simulink model "model_only_GD_constant_muscle_admittance_aug_gain"  (R2020a)
settings: Solver=FixedStepAuto  StartTime=0.0  StopTime=180  FixedStep=0.002  RelTol=1e-6  EnableMultiTasking=on
libraries: dspmtrx3 x1
settings Model: SimulationMode=accelerator  Creator=Tenghu  LastModifiedBy=ripme
settings DataIOCC: SaveFormat=Array  SignalLoggingSaveFormat=ModelDataLogs  SaveOutput=off  ReturnWorkspaceOutputs=off
settings OptimizationCC: ExpressionDepthLimit=2147483647  EfficientMapNaN2IntZero=off  LifeSpan=inf
settings DebuggingCC: UnderspecifiedInitializationDetection=Classic  MergeDetectMultiDrivingBlocksExec=none  SolverPrmCheckMsg=warning  FcnCallInpInsideContextMsg=warning  StateNameClashWarn=warning  SFUnexpectedBacktrackingDiag=warning  SFNoUnconditionalDefaultTransitionDiag=warning  SFExecutionAtInitializationDiag=none  UnderSpecifiedDimensionMsg=warning  ArithmeticOperatorsInVariantConditions=warning
settings HardwareCC: ProdBitPerPointer=32  ProdBitPerSizeT=32  ProdBitPerPtrDiffT=32  ProdLargestAtomicFloat=None  ProdIntDivRoundTo=Undefined  ProdEndianess=Unspecified  ProdWordSize=32  ProdHWDeviceType=32-bit Generic  TargetBitPerPointer=64  TargetBitPerSizeT=64  TargetBitPerPtrDiffT=64  TargetLongLongMode=on  TargetIntDivRoundTo=Zero  TargetEndianess=LittleEndian  TargetWordSize=64  TargetHWDeviceType=MATLAB Host  ProdEqTarget=off
settings ModelReferenceCC: PropagateSignalLabelsOutOfModel=off
settings SFSimCC: SimUseLocalCustomCode=off  SimParseCustomCode=off  CustomCodeUndefinedFunction=UseInterfaceOnly
settings CodeAppCC: MaxIdLength=128
settings GRTTargetCC: TargetLangStandard=C89/C90 (ANSI)  CombineOutputUpdateFcns=off  GRTInterface=on
settings ConfigComp: CovMetricSettings=dw  CovHtmlReporting=on  CovSaveCumulativeToWorkspaceVar=on  CovSaveSingleToWorkspaceVar=on  CovExternalEMLEnable=off

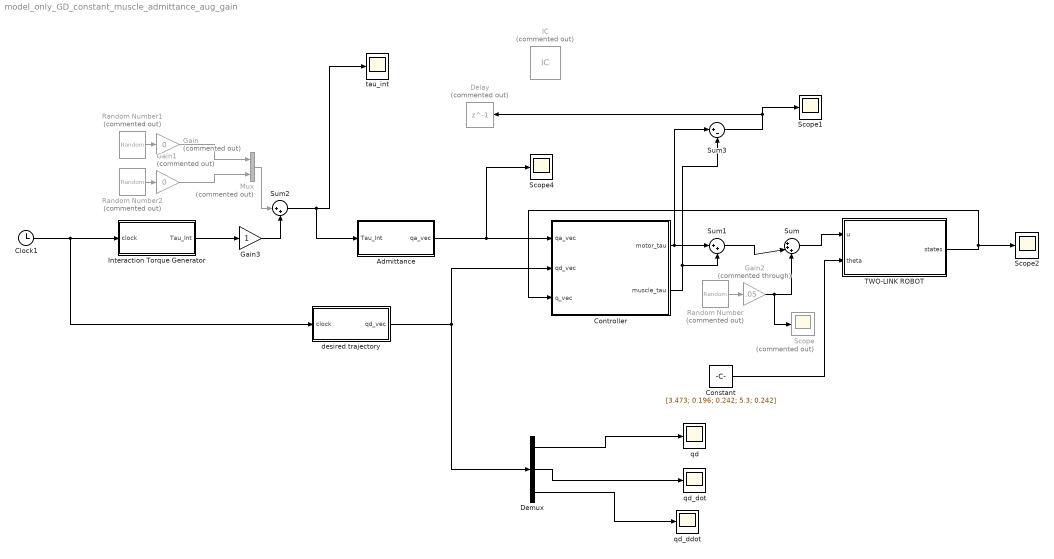
== system model_only_GD_constant_muscle_admittance_aug_gain ==
  Admittance : Subsystem
  Clock1 : Clock
  Constant : Constant  Value=|
      | [3.473;
      | 0.196;
      | 0.242; 5.3; 0.242]
  Controller : Subsystem
  Delay : Delay  Commented=on  DelayLength=1  InitialCondition=[0;0]
  Demux : Demux  Outputs=3
  Gain : Gain  Commented=on  Gain=0
  Gain1 : Gain  Commented=on  Gain=0
  Gain2 : Gain  Commented=through  Gain=.05
  Gain3 : Gain
  IC : InitialCondition  Commented=on  Value=[0;0]
  Interaction Torque Generator : Subsystem
  Mux : Mux  Commented=on  Inputs=2
  Random Number : RandomNumber  Commented=on  Mean=5  SampleTime=0.002
  Random Number1 : RandomNumber  Commented=on  Mean=1  Variance=.5  SampleTime=0.002
  Random Number2 : RandomNumber  Commented=on  Mean=1  Variance=.2  SampleTime=0.002
  Scope : Scope  Commented=on
  Scope1 : Scope
  Scope2 : Scope
  Scope4 : Scope
  Sum : Sum  Inputs=|+++
  Sum1 : Sum  Inputs=|++
  Sum2 : Sum  Inputs=|++
  Sum3 : Sum  Inputs=|+-
  TWO-LINK ROBOT : Subsystem
  desired trajectory : Subsystem
  qd : Scope
  qd_ddot : Scope
  qd_dot : Scope
  tau_int : Scope
  wires:
  TWO-LINK ROBOT/1(states) -> Scope2/1, Controller/3(q_vec)
  Sum/1 -> TWO-LINK ROBOT/1(u)
  Clock1/1 -> Interaction Torque Generator/1(clock), desired trajectory/1(clock)
  desired trajectory/1(qd_vec) -> Controller/2(qd_vec), Demux/1
  Admittance/1(qa_vec) -> Scope4/1, Controller/1(qa_vec)
  Controller/1(motor_tau) -> Sum3/1, Sum1/1
  Sum1/1 -> Sum/2
  Sum2/1 -> Admittance/1("Tau_Int "), tau_int/1
  Mux/1 -> Sum2/1
  Random Number1/1 -> Gain/1
  Random Number2/1 -> Gain1/1
  Gain1/1 -> Mux/2
  Gain/1 -> Mux/1
  Random Number/1 -> Gain2/1
  Gain2/1 -> Sum/3, Scope/1
  Controller/2(muscle_tau) -> Sum1/2, Sum3/2
  Sum3/1 -> Scope1/1, Delay/1
  Gain3/1 -> Sum2/2
  Interaction Torque Generator/1(Tau_Int) -> Gain3/1
  Demux/1 -> qd/1
  Demux/2 -> qd_dot/1
  Demux/3 -> qd_ddot/1
  Constant/1 -> TWO-LINK ROBOT/2(theta)

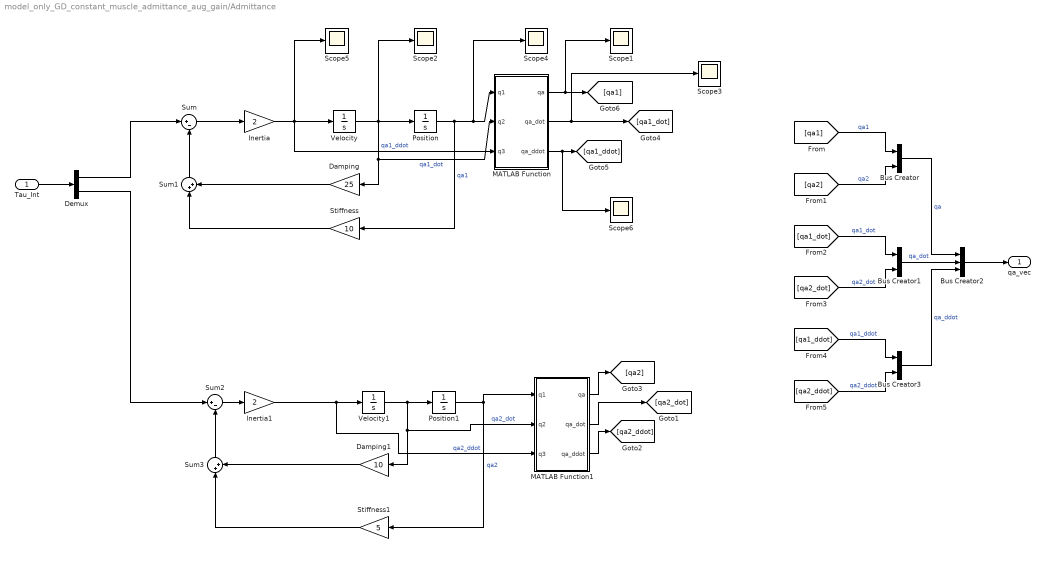
== system model_only_GD_constant_muscle_admittance_aug_gain/Admittance ==
  "Tau_Int " : Inport
  Bus Creator : BusCreator  Inputs=2
  Bus Creator1 : BusCreator  Inputs=2
  Bus Creator2 : BusCreator  Inputs=3
  Bus Creator3 : BusCreator  Inputs=2
  Damping : Gain  Gain=25
  Damping1 : Gain  Gain=10
  Demux : Demux  Outputs=2
  Inertia : Gain  Gain=2
  Inertia1 : Gain  Gain=2
  MATLAB Function : MATLAB Function  TreatAsAtomicUnit=on
  MATLAB Function1 : MATLAB Function  TreatAsAtomicUnit=on
  Position : Integrator
  Position1 : Integrator
  Scope{1..6} (6 alike) : Scope
  Stiffness : Gain  Gain=10
  Stiffness1 : Gain  Gain=5
  Sum : Sum  Inputs=|+-
  Sum1 : Sum  Inputs=|++
  Sum2 : Sum  Inputs=|+-
  Sum3 : Sum  Inputs=|++
  Velocity : Integrator
  Velocity1 : Integrator
  qa_vec : Outport  VectorParamsAs1DForOutWhenUnconnected=off
  wires:
  Inertia/1 -> MATLAB Function/3(q3), Scope5/1, Velocity/1  "qa1_ddot"
  Sum/1 -> Inertia/1
  Sum1/1 -> Sum/2
  Velocity/1 -> MATLAB Function/2(q2), Damping/1, Scope2/1, Position/1  "qa1_dot"
  Damping/1 -> Sum1/2
  Stiffness/1 -> Sum1/1
  Position/1 -> Scope4/1, MATLAB Function/1(q1), Stiffness/1  "qa1"
  "Tau_Int "/1 -> Demux/1
  Demux/1 -> Sum/1
  Velocity1/1 -> Position1/1, MATLAB Function1/2(q2), Damping1/1  "qa2_dot"
  Inertia1/1 -> MATLAB Function1/3(q3), Velocity1/1  "qa2_ddot"
  Position1/1 -> MATLAB Function1/1(q1), Stiffness1/1  "qa2"
  Sum2/1 -> Inertia1/1
  Damping1/1 -> Sum3/2
  Demux/2 -> Sum2/1
  Sum3/1 -> Sum2/2
  Stiffness1/1 -> Sum3/1
  [qa1] -> Bus Creator/1  "qa1"
  [qa2] -> Bus Creator/2  "qa2"
  [qa1_dot] -> Bus Creator1/1  "qa1_dot"
  [qa2_dot] -> Bus Creator1/2  "qa2_dot"
  Bus Creator1/1 -> Bus Creator2/2  "qa_dot"
  Bus Creator/1 -> Bus Creator2/1  "qa"
  [qa1_ddot] -> Bus Creator3/1  "qa1_ddot"
  [qa2_ddot] -> Bus Creator3/2  "qa2_ddot"
  Bus Creator3/1 -> Bus Creator2/3  "qa_ddot"
  Bus Creator2/1 -> qa_vec/1
  MATLAB Function/1(qa) -> Scope1/1, [qa1]
  MATLAB Function/2(qa_dot) -> [qa1_dot], Scope3/1
  MATLAB Function/3(qa_ddot) -> Scope6/1, [qa1_ddot]
  MATLAB Function1/1(qa) -> [qa2]
  MATLAB Function1/3(qa_ddot) -> [qa2_ddot]
  MATLAB Function1/2(qa_dot) -> [qa2_dot]

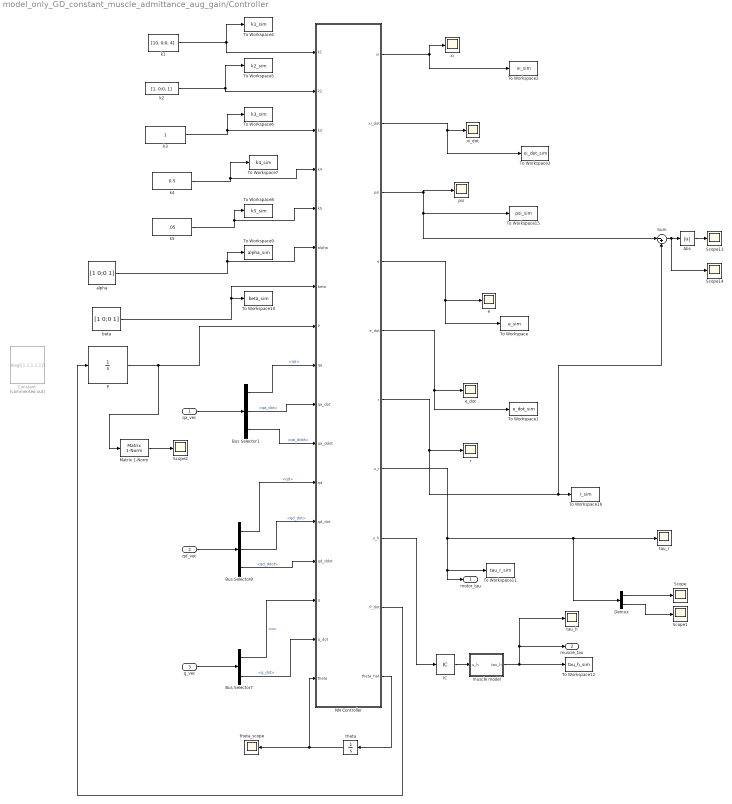
== system model_only_GD_constant_muscle_admittance_aug_gain/Controller ==
  qa_vec : Inport
  qd_vec : Inport  Port=2
  q_vec : Inport  Port=3
  Abs : Abs
  Bus Selector1 : BusSelector  OutputSignals=qa,qa_dot,qa_ddot
  Bus Selector7 : BusSelector  OutputSignals=q,q_dot
  Bus Selector8 : BusSelector  OutputSignals=qd,qd_dot,qd_ddot
  Constant : Constant  Commented=on  Value=diag([1,1,1,1,1])
  Demux : Demux  Outputs=2
  IC : InitialCondition  Value=[0;0]
  Matrix 1-Norm : dspmtrx3/Matrix  1-Norm  roundingMode=Floor  overflowMode=off  outputDataTypeStr=Inherit: Same as accumulator  outputMin=[]  outputMax=[]  outputLastDataTypeStr=Inherit: Same as accumulator
      settings: SourceProductBaseCode=DS
  "NN Controller " : MATLAB Function  TreatAsAtomicUnit=on
  P : Integrator  InitialCondition=diag([1,1,1,1,1]*5)
  Scope{,1..2,13..14} (5 alike) : Scope
  Sum : Sum  Inputs=|-+
  To Workspace : ToWorkspace  VariableName=e_sim  SaveFormat=Timeseries  SampleTime=-1
  To Workspace1 : ToWorkspace  VariableName=e_dot_sim  SaveFormat=Timeseries  SampleTime=-1
  To Workspace10 : ToWorkspace  VariableName=beta_sim  SaveFormat=Timeseries  SampleTime=-1
      settings: MaxDataPoints=1
  To Workspace11 : ToWorkspace  VariableName=tau_r_sim  SaveFormat=Timeseries  SampleTime=-1
  To Workspace12 : ToWorkspace  VariableName=tau_h_sim  SaveFormat=Timeseries  SampleTime=-1
  To Workspace15 : ToWorkspace  VariableName=psi_sim  SaveFormat=Timeseries  SampleTime=-1
  To Workspace16 : ToWorkspace  VariableName=r_sim  SaveFormat=Timeseries  SampleTime=-1
  To Workspace2 : ToWorkspace  VariableName=xi_sim  SaveFormat=Timeseries  SampleTime=-1
  To Workspace3 : ToWorkspace  VariableName=xi_dot_sim  SaveFormat=Timeseries  SampleTime=-1
  To Workspace4 : ToWorkspace  VariableName=k1_sim  SaveFormat=Timeseries  SampleTime=-1
      settings: MaxDataPoints=1
  To Workspace5 : ToWorkspace  VariableName=k2_sim  SaveFormat=Timeseries  SampleTime=-1
      settings: MaxDataPoints=1
  To Workspace6 : ToWorkspace  VariableName=k3_sim  SaveFormat=Timeseries  SampleTime=-1
      settings: MaxDataPoints=1
  To Workspace7 : ToWorkspace  VariableName=k4_sim  SaveFormat=Timeseries  SampleTime=-1
      settings: MaxDataPoints=1
  To Workspace8 : ToWorkspace  VariableName=k5_sim  SaveFormat=Timeseries  SampleTime=-1
      settings: MaxDataPoints=1
  To Workspace9 : ToWorkspace  VariableName=alpha_sim  SaveFormat=Timeseries  SampleTime=-1
      settings: MaxDataPoints=1
  alpha : Constant  Value=[1 0;0 1]
  beta : Constant  Value=[1 0;0 1]
  e : Scope
  e_dot : Scope
  "k1 " : Constant  Value=[10, 0;0, 4]  VectorParams1D=off
  k2 : Constant  Value=[1, 0;0, 1]
  k3 : Constant
  k4 : Constant  Value=0.5
  k5 : Constant  Value=.05
  muscle model : MATLAB Function  TreatAsAtomicUnit=on
  "psi " : Scope
  r : Scope
  tau_h : Scope
  tau_r : Scope
  theta : Integrator  InitialCondition=[1;1;1;1;1]
  theta_scope : Scope
  xi : Scope
  xi_dot : Scope
  motor_tau : Outport  VectorParamsAs1DForOutWhenUnconnected=off
  muscle_tau : Outport  Port=2  VectorParamsAs1DForOutWhenUnconnected=off
  wires:
  q_vec/1 -> Bus Selector7/1
  qd_vec/1 -> Bus Selector8/1
  qa_vec/1 -> Bus Selector1/1
  "k1 "/1 -> To Workspace4/1, "NN Controller "/1(k1)
  k2/1 -> To Workspace5/1, "NN Controller "/2(k2)
  k3/1 -> To Workspace6/1, "NN Controller "/3(k3)
  k4/1 -> To Workspace7/1, "NN Controller "/4(k4)
  k5/1 -> To Workspace8/1, "NN Controller "/5(k5)
  beta/1 -> To Workspace10/1, "NN Controller "/7(beta)
  alpha/1 -> To Workspace9/1, "NN Controller "/6(alpha)
  Bus Selector1/2 -> "NN Controller "/10(qa_dot)  "<qa_dot>"
  Bus Selector1/1 -> "NN Controller "/9(qa)  "<qa>"
  Bus Selector1/3 -> "NN Controller "/11(qa_ddot)  "<qa_ddot>"
  Bus Selector7/1 -> "NN Controller "/15(q)  "<q>"
  Bus Selector7/2 -> "NN Controller "/16(q_dot)  "<q_dot>"
  Bus Selector8/1 -> "NN Controller "/12(qd)  "<qd>"
  Bus Selector8/2 -> "NN Controller "/13(qd_dot)  "<qd_dot>"
  Bus Selector8/3 -> "NN Controller "/14(qd_ddot)  "<qd_ddot>"
  "NN Controller "/1(xi) -> To Workspace2/1, xi/1
  "NN Controller "/2(xi_dot) -> To Workspace3/1, xi_dot/1
  "NN Controller "/5(e_dot) -> To Workspace1/1, e_dot/1
  "NN Controller "/3(psi) -> Sum/1, To Workspace15/1, "psi "/1
  "NN Controller "/6(r) -> Sum/2, To Workspace16/1, r/1
  Sum/1 -> Scope14/1, Abs/1
  Abs/1 -> Scope13/1
  "NN Controller "/7(u_r) -> motor_tau/1, To Workspace11/1, Demux/1, tau_r/1
  "NN Controller "/8(u_h) -> IC/1
  muscle model/1(tau_h) -> tau_h/1, muscle_tau/1, To Workspace12/1
  "NN Controller "/4(e) -> To Workspace/1, e/1
  Demux/1 -> Scope/1
  Demux/2 -> Scope1/1
  "NN Controller "/10(theta_hat) -> theta/1
  theta/1 -> "NN Controller "/17(theta), theta_scope/1
  IC/1 -> muscle model/1(u_h)
  P/1 -> Matrix 1-Norm/1, "NN Controller "/8(P)
  "NN Controller "/9(P_dot) -> P/1
  Matrix 1-Norm/1 -> Scope2/1

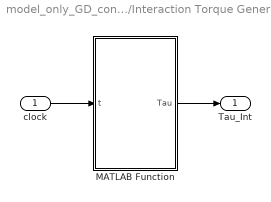
== system model_only_GD_constant_muscle_admittance_aug_gain/Interaction Torque Generator ==
  clock : Inport
  MATLAB Function : MATLAB Function  TreatAsAtomicUnit=on
  Tau_Int : Outport  VectorParamsAs1DForOutWhenUnconnected=off
  wires:
  MATLAB Function/1(Tau) -> Tau_Int/1
  clock/1 -> MATLAB Function/1(t)

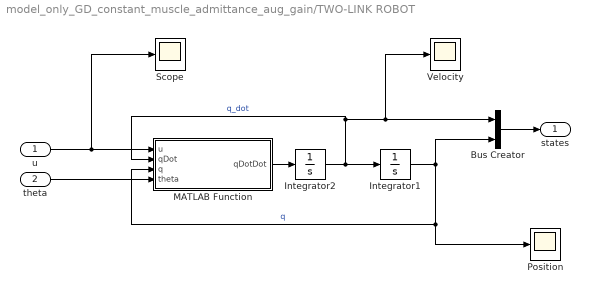
== system model_only_GD_constant_muscle_admittance_aug_gain/TWO-LINK ROBOT ==
  u : Inport
  theta : Inport  Port=2
  Bus Creator : BusCreator  Inputs=2
  Integrator1 : Integrator  InitialCondition=[0;0]
  Integrator2 : Integrator  InitialCondition=[1;2]
  MATLAB Function : MATLAB Function  TreatAsAtomicUnit=on
  Position : Scope
  Scope : Scope
  Velocity : Scope
  states : Outport  VectorParamsAs1DForOutWhenUnconnected=off
  wires:
  u/1 -> Scope/1, MATLAB Function/1(u)
  Integrator1/1 -> Bus Creator/2, Position/1, MATLAB Function/3(q)  "q"
  Integrator2/1 -> Velocity/1, Bus Creator/1, MATLAB Function/2(qDot), Integrator1/1  "q_dot"
  Bus Creator/1 -> states/1
  MATLAB Function/1(qDotDot) -> Integrator2/1
  theta/1 -> MATLAB Function/4(theta)

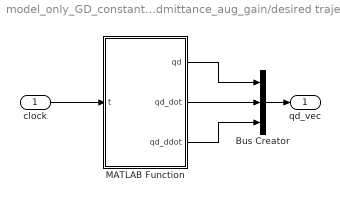
== system model_only_GD_constant_muscle_admittance_aug_gain/desired trajectory ==
  clock : Inport
  Bus Creator : BusCreator  Inputs=3
  MATLAB Function : MATLAB Function  TreatAsAtomicUnit=on
  qd_vec : Outport  VectorParamsAs1DForOutWhenUnconnected=off
  wires:
  clock/1 -> MATLAB Function/1(t)
  MATLAB Function/3(qd_ddot) -> Bus Creator/3
  MATLAB Function/2(qd_dot) -> Bus Creator/2
  MATLAB Function/1(qd) -> Bus Creator/1
  Bus Creator/1 -> qd_vec/1

== matlab function model_only_GD_constant_muscle_admittance_aug_gain/desired trajectory/MATLAB Function ==
  data: qd output; qd_dot output; qd_ddot output; t input
function [qd,qd_dot,qd_ddot]  = des_trajectory(t)
%#codegen

% This block supports an embeddable subset of the MATLAB language.
% See the help menu for details. 

qd1=-cos(t)+.95;
qd2=sin(0.5*t);

qd1_dot=sin(t);
qd2_dot=0.5*cos(0.5*t);

qd1_ddot = cos(t);
qd2_ddot = -0.25*sin(0.5*t);

qd=[qd1;qd2];
qd_dot = [qd1_dot;qd2_dot];
qd_ddot = [qd1_ddot; qd2_ddot];

end

== matlab function model_only_GD_constant_muscle_admittance_aug_gain/Interaction Torque Generator/MATLAB Function ==
  data: t input; Tau output
function Tau   = TauInt(t)
%#codegen

% This block supports an embeddable subset of the MATLAB language.
% See the help menu for details. 

tau1=3*sin(.4*t);
tau2=2*sin(.6*t);

Tau = [tau1;tau2];
end

== matlab function model_only_GD_constant_muscle_admittance_aug_gain/Controller/muscle model ==
  data: u_h input; tau_h output
function tau_h = fcn(u_h)

if u_h(1)>0
    s_k1 = 1;
    s_k2 = 0;
else
    s_k1 = 0;
    s_k2 = 1;
end

if u_h(2)>0
    s_c1 = 1;
    s_c2 = 0;
else
    s_c1 = 0;
    s_c2 = 1;
end

SIGMA = [s_k1 0;
         s_k2 0;
         0 s_c1;
         0 s_c2];
     
B_bi = .7;
B_tri = .6;
B_flex = .4;
B_ext = .3;
     
B_h = [B_bi B_tri 0 0;
       0 0 B_flex B_ext];

u = [20*tanh(1/20*u_h(1));
     12*tanh(1/12*u_h(2))];

tau_h = B_h*SIGMA*u;

== matlab function model_only_GD_constant_muscle_admittance_aug_gain/TWO-LINK ROBOT/MATLAB Function ==
  data: u input; qDot input; q input; qDotDot output; theta input
function qDotDot = dynamics(u,qDot,q, theta)
%#codegen

p1 = theta(1);
p2 = theta(2);
p3 = theta(3);

fd1 = theta(4);
fd2 = theta(5);

M = [p1+(2*p2*cos(q(2))), p3+(2*p2*cos(q(2))); p3+(2*p2*cos(q(2))), p3];
Vm = [-p2*sin(q(2))*qDot(2), -p2*sin(q(2))*(qDot(1)+qDot(2)); -p2*sin(q(2))*(qDot(2)-qDot(1)), 0];
Fd = [fd1, 0; 0, fd2];

qDotDot = M\(u - Vm*qDot - Fd*qDot);

end

== matlab function model_only_GD_constant_muscle_admittance_aug_gain/Admittance/MATLAB Function ==
  data: q1 input; qa output; qa_dot output; qa_ddot output; q2 input; q3 input
function [qa,qa_dot,qa_ddot] = fcn(q1,q2,q3)

qa = tanh(q1);
qa_dot = q2*sech(q1)^2;
qa_ddot = -2*q2*tanh(q1)*sech(q1)^2+q3*sech(q1)^2;

end

== matlab function model_only_GD_constant_muscle_admittance_aug_gain/Admittance/MATLAB Function1 ==
  data: q1 input; qa output; qa_dot output; qa_ddot output; q2 input; q3 input
function [qa,qa_dot,qa_ddot] = fcn(q1,q2,q3)

qa = tanh(q1);
qa_dot = q2*sech(q1)^2;
qa_ddot = -2*q2*tanh(q1)*sech(q1)^2+q3*sech(q1)^2;

end

== matlab function model_only_GD_constant_muscle_admittance_aug_gain/Controller/NN Controller  ==
  data: k1 input; xi output; xi_dot output; psi output; e output size=2; e_dot output; r output; u_r output; u_h output; P_dot output; k2 input; k3 input; k4 input; k5 input; alpha input; beta input; P input; qa input; qa_dot input; qa_ddot input; qd input; qd_dot input; qd_ddot input; q input; q_dot input; theta input; theta_hat output
function [xi,xi_dot,psi,e,e_dot,r,u_r,u_h,P_dot, theta_hat] = controller(k1,k2,k3,k4,k5,alpha,beta,P,qa,qa_dot,qa_ddot,qd,qd_dot,qd_ddot,q,q_dot, theta)
%#codegen

%% Error Systems
xi=qa + qd - q; 
xi_dot = qa_dot + qd_dot - q_dot;
psi = xi_dot + beta*xi; 

zeta = [xi' psi']';
phi = [qa' qa_dot' qa_ddot']';

e = qd - q;
e_dot = qd_dot - q_dot;
r = e_dot + alpha*e;

z = [e' r']';
%set up the graient descent
eta = (qa_ddot+qd_ddot+beta*xi_dot);
Y_M = [eta(1), 2*cos(q(2))*(eta(1)+eta(2)), eta(2), 0, 0; 0, 2*cos(q(2))*eta(1), eta(2), 0, 0];

chi = (qa_dot+qd_dot+beta*xi);
Y_C = -sin(q(2))*[0, (q_dot(2)*chi(1))+((q_dot(1)+q_dot(2))*chi(2)), 0, 0, 0; 0, (q_dot(2)-q_dot(1))*chi(1), 0, 0, 0];

Y_b = [0, 0, 0, q_dot(1), 0; 0, 0, 0, 0, q_dot(2)];

Y1 = Y_M+Y_C+Y_b;

%u_r=k1*r+([1;1]*(k2+k3*norm(r)+k4*norm(r)^2));
u_r=k1*psi+Y1*theta;%+(sign(psi)*(k2+k3*norm(psi)+k4*norm(psi)^2));


Br=1;
% Motor Controller
%square = sign(psi)*(k3*norm(zeta)^2+k4*norm(phi)+k5*norm(phi)^2);
%tau_r = 100*tanh(1/100*tau_r);
% Muscle Controller
B_min=1;
%u_h = 1/B_min*(k2*r);
%u_h=[1;1];
u_h=k5*r;
%tau_h = 10*tanh(1/10*tau_h);
P_dot = -P'*Y1'*Y1*P;
theta_hat = P*Y1'*psi;
end
